simulink library "vst"  (Simulink 8.1)
settings: Solver=ode45  StartTime=0.0  StopTime=10.0  RelTol=1e-3
undefined symbols (not defined in the file or in its folder): ENUM_EMSOPSTATE_NORMAL, ENUM_TCMFAULTSTATE_NORMAL
settings Model: Creator=xsellart  LastModifiedBy=AT015555

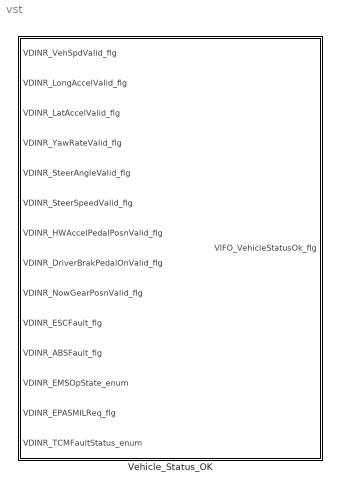
== system vst ==
  Vehicle_Status_OK : Subsystem

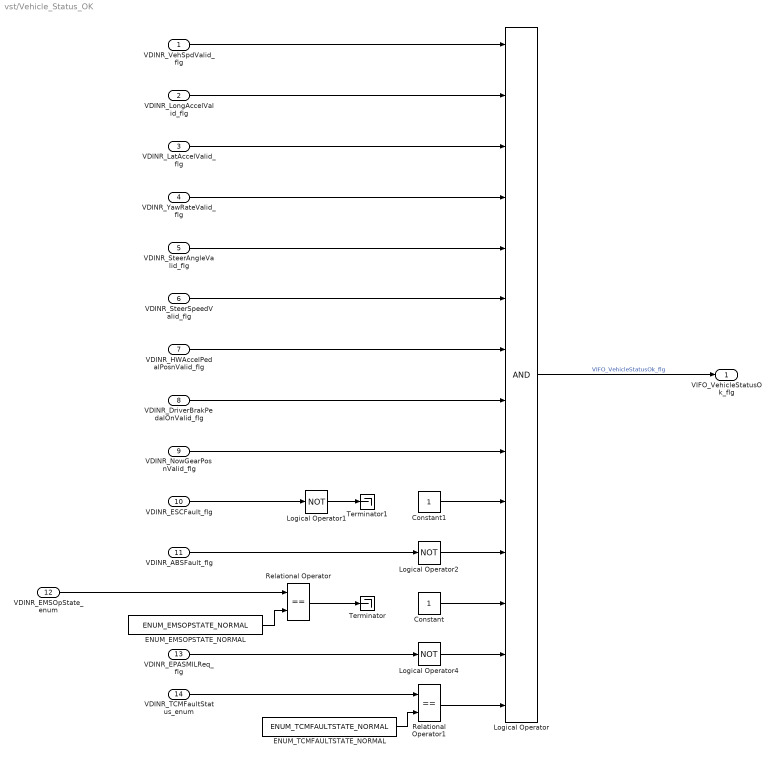
== system vst/Vehicle_Status_OK ==
  "VDINR_VehSpdValid_flg " : Inport
  "VDINR_LongAccelValid_flg " : Inport  Port=2
  "VDINR_LatAccelValid_flg " : Inport  Port=3
  "VDINR_YawRateValid_flg " : Inport  Port=4
  "VDINR_SteerAngleValid_flg " : Inport  Port=5
  "VDINR_SteerSpeedValid_flg " : Inport  Port=6
  "VDINR_HWAccelPedalPosnValid_flg " : Inport  Port=7
  "VDINR_DriverBrakPedalOnValid_flg " : Inport  Port=8
  "VDINR_NowGearPosnValid_flg " : Inport  Port=9
  "VDINR_ESCFault_flg " : Inport  Port=10
  "VDINR_ABSFault_flg " : Inport  Port=11
  "VDINR_EMSOpState_enum " : Inport  Port=12
  "VDINR_EPASMILReq_flg " : Inport  Port=13
  "VDINR_TCMFaultStatus_enum " : Inport  Port=14
  Constant : Constant
  Constant1 : Constant  OutDataTypeStr=boolean
  ENUM_EMSOPSTATE_NORMAL : Constant  Value=ENUM_EMSOPSTATE_NORMAL
  ENUM_TCMFAULTSTATE_NORMAL : Constant  Value=ENUM_TCMFAULTSTATE_NORMAL
  Logical Operator : Logic  Inputs=14  AllPortsSameDT=off  OutDataTypeStr=boolean
  Logical Operator1 : Logic  Operator=NOT  AllPortsSameDT=off  OutDataTypeStr=boolean
  Logical Operator2 : Logic  Operator=NOT  AllPortsSameDT=off  OutDataTypeStr=boolean
  Logical Operator4 : Logic  Operator=NOT  AllPortsSameDT=off  OutDataTypeStr=boolean
  Relational Operator : RelationalOperator  Operator===  OutDataTypeStr=boolean
  Relational Operator1 : RelationalOperator  Operator===  OutDataTypeStr=boolean
  Terminator : Terminator
  Terminator1 : Terminator
  VIFO_VehicleStatusOk_flg : Outport
  wires:
  "VDINR_VehSpdValid_flg "/1 -> Logical Operator/1
  "VDINR_LongAccelValid_flg "/1 -> Logical Operator/2
  "VDINR_LatAccelValid_flg "/1 -> Logical Operator/3
  "VDINR_YawRateValid_flg "/1 -> Logical Operator/4
  "VDINR_SteerAngleValid_flg "/1 -> Logical Operator/5
  "VDINR_SteerSpeedValid_flg "/1 -> Logical Operator/6
  "VDINR_HWAccelPedalPosnValid_flg "/1 -> Logical Operator/7
  "VDINR_DriverBrakPedalOnValid_flg "/1 -> Logical Operator/8
  "VDINR_NowGearPosnValid_flg "/1 -> Logical Operator/9
  Logical Operator/1 -> VIFO_VehicleStatusOk_flg/1  "VIFO_VehicleStatusOk_flg"
  "VDINR_ESCFault_flg "/1 -> Logical Operator1/1
  Logical Operator1/1 -> Terminator1/1
  Logical Operator2/1 -> Logical Operator/11
  Logical Operator4/1 -> Logical Operator/13
  "VDINR_ABSFault_flg "/1 -> Logical Operator2/1
  "VDINR_EPASMILReq_flg "/1 -> Logical Operator4/1
  "VDINR_EMSOpState_enum "/1 -> Relational Operator/1
  ENUM_EMSOPSTATE_NORMAL/1 -> Relational Operator/2
  Relational Operator/1 -> Terminator/1
  Relational Operator1/1 -> Logical Operator/14
  ENUM_TCMFAULTSTATE_NORMAL/1 -> Relational Operator1/2
  "VDINR_TCMFaultStatus_enum "/1 -> Relational Operator1/1
  Constant/1 -> Logical Operator/12
  Constant1/1 -> Logical Operator/10
